simulink model "Sim118Bus"  (R2020b)
(part 2 of 2)

  Branch2-12/RConn1 -- Bus12/RConn1 -- Branch12-12/LConn1 -- Branch12-117/LConn1 -- Branch12-16/LConn1 -- Branch12-14/LConn1 -- Branch11-12/RConn1 -- Branch7-12/RConn1 -- Branch3-12/RConn1
  Branch2-12/RConn2 -- Bus12/RConn2 -- Branch12-12/LConn2 -- Branch12-117/LConn2 -- Branch12-16/LConn2 -- Branch12-14/LConn2 -- Branch11-12/RConn2 -- Branch7-12/RConn2 -- Branch3-12/RConn2
  Branch2-12/RConn3 -- Bus12/RConn3 -- Branch12-12/LConn3 -- Branch12-117/LConn3 -- Branch12-16/LConn3 -- Branch12-14/LConn3 -- Branch11-12/RConn3 -- Branch7-12/RConn3 -- Branch3-12/RConn3
  Branch2-12/LConn1 -- Bus2/RConn1 -- Branch2-2/LConn1 -- Branch2-69/LConn1
  Branch2-12/LConn2 -- Bus2/RConn2 -- Branch2-2/LConn2 -- Branch2-69/LConn2
  Branch2-12/LConn3 -- Bus2/RConn3 -- Branch2-2/LConn3 -- Branch2-69/LConn3
  Branch2-69/RConn1 -- Bus69/RConn1 -- Branch69-69/LConn1 -- Branch3-69/RConn1
  Branch2-69/RConn2 -- Bus69/RConn2 -- Branch69-69/LConn2 -- Branch3-69/RConn2
  Branch2-69/RConn3 -- Bus69/RConn3 -- Branch69-69/LConn3 -- Branch3-69/RConn3
  Branch3-5/RConn1 -- Bus5/RConn1 -- Branch5-5/LConn1 -- Branch5-11/LConn1 -- Transformer5-8/LConn1 -- Branch5-6/LConn1 -- Branch4-5/RConn1
  Branch3-5/RConn2 -- Bus5/RConn2 -- Branch5-5/LConn2 -- Branch5-11/LConn2 -- Transformer5-8/LConn2 -- Branch5-6/LConn2 -- Branch4-5/RConn2
  Branch3-5/RConn3 -- Bus5/RConn3 -- Branch5-5/LConn3 -- Branch5-11/LConn3 -- Transformer5-8/LConn3 -- Branch5-6/LConn3 -- Branch4-5/RConn3
  Branch3-5/LConn1 -- Bus3/RConn1 -- Branch3-3/LConn1 -- Branch3-69/LConn1 -- Branch3-12/LConn1
  Branch3-5/LConn2 -- Bus3/RConn2 -- Branch3-3/LConn2 -- Branch3-69/LConn2 -- Branch3-12/LConn2
  Branch3-5/LConn3 -- Bus3/RConn3 -- Branch3-3/LConn3 -- Branch3-69/LConn3 -- Branch3-12/LConn3
  Branch4-5/LConn1 -- Bus4/RConn1 -- Branch4-4/LConn1 -- Branch4-11/LConn1
  Branch4-5/LConn2 -- Bus4/RConn2 -- Branch4-4/LConn2 -- Branch4-11/LConn2
  Branch4-5/LConn3 -- Bus4/RConn3 -- Branch4-4/LConn3 -- Branch4-11/LConn3
  Branch4-11/RConn1 -- Bus11/RConn1 -- Branch11-11/LConn1 -- Branch11-13/LConn1 -- Branch11-12/LConn1 -- Branch5-11/RConn1
  Branch4-11/RConn2 -- Bus11/RConn2 -- Branch11-11/LConn2 -- Branch11-13/LConn2 -- Branch11-12/LConn2 -- Branch5-11/RConn2
  Branch4-11/RConn3 -- Bus11/RConn3 -- Branch11-11/LConn3 -- Branch11-13/LConn3 -- Branch11-12/LConn3 -- Branch5-11/RConn3
  Branch5-6/RConn1 -- Bus6/RConn1 -- Branch6-6/LConn1 -- Branch6-7/LConn1
  Branch5-6/RConn2 -- Bus6/RConn2 -- Branch6-6/LConn2 -- Branch6-7/LConn2
  Branch5-6/RConn3 -- Bus6/RConn3 -- Branch6-6/LConn3 -- Branch6-7/LConn3
  Branch5-8/RConn1 -- Bus8/RConn1 -- Branch8-8/LConn1 -- Branch8-30/LConn1 -- Branch8-9/LConn1
  Branch5-8/RConn2 -- Bus8/RConn2 -- Branch8-8/LConn2 -- Branch8-30/LConn2 -- Branch8-9/LConn2
  Branch5-8/RConn3 -- Bus8/RConn3 -- Branch8-8/LConn3 -- Branch8-30/LConn3 -- Branch8-9/LConn3
  Transformer5-8/RConn1 -- Branch5-8/LConn1
  Transformer5-8/RConn2 -- Branch5-8/LConn2
  Transformer5-8/RConn3 -- Branch5-8/LConn3
  Branch6-7/RConn1 -- Bus7/RConn1 -- Branch7-7/LConn1 -- Branch7-12/LConn1
  Branch6-7/RConn2 -- Bus7/RConn2 -- Branch7-7/LConn2 -- Branch7-12/LConn2
  Branch6-7/RConn3 -- Bus7/RConn3 -- Branch7-7/LConn3 -- Branch7-12/LConn3
  Branch8-9/RConn1 -- Bus9/RConn1 -- Branch9-9/LConn1 -- Branch9-10/LConn1
  Branch8-9/RConn2 -- Bus9/RConn2 -- Branch9-9/LConn2 -- Branch9-10/LConn2
  Branch8-9/RConn3 -- Bus9/RConn3 -- Branch9-9/LConn3 -- Branch9-10/LConn3
  Branch8-30/RConn1 -- Bus30/RConn1 -- Branch30-30/LConn1 -- Branch30-38/LConn1 -- Branch26-30/RConn1 -- Branch17-30/RConn1
  Branch8-30/RConn2 -- Bus30/RConn2 -- Branch30-30/LConn2 -- Branch30-38/LConn2 -- Branch26-30/RConn2 -- Branch17-30/RConn2
  Branch8-30/RConn3 -- Bus30/RConn3 -- Branch30-30/LConn3 -- Branch30-38/LConn3 -- Branch26-30/RConn3 -- Branch17-30/RConn3
  Branch9-10/RConn1 -- Bus10/RConn1 -- Branch10-10/LConn1
  Branch9-10/RConn2 -- Bus10/RConn2 -- Branch10-10/LConn2
  Branch9-10/RConn3 -- Bus10/RConn3 -- Branch10-10/LConn3
  Branch11-13/RConn1 -- Bus13/RConn1 -- Branch13-13/LConn1 -- Branch13-15/LConn1
  Branch11-13/RConn2 -- Bus13/RConn2 -- Branch13-13/LConn2 -- Branch13-15/LConn2
  Branch11-13/RConn3 -- Bus13/RConn3 -- Branch13-13/LConn3 -- Branch13-15/LConn3
  Branch12-14/RConn1 -- Bus14/RConn1 -- Branch14-14/LConn1 -- Branch14-15/LConn1
  Branch12-14/RConn2 -- Bus14/RConn2 -- Branch14-14/LConn2 -- Branch14-15/LConn2
  Branch12-14/RConn3 -- Bus14/RConn3 -- Branch14-14/LConn3 -- Branch14-15/LConn3
  Branch12-16/RConn1 -- Bus16/RConn1 -- Branch16-16/LConn1 -- Branch16-17/LConn1
  Branch12-16/RConn2 -- Bus16/RConn2 -- Branch16-16/LConn2 -- Branch16-17/LConn2
  Branch12-16/RConn3 -- Bus16/RConn3 -- Branch16-16/LConn3 -- Branch16-17/LConn3
  Branch12-117/RConn1 -- Bus117/RConn1 -- Branch117-117/LConn1
  Branch12-117/RConn2 -- Bus117/RConn2 -- Branch117-117/LConn2
  Branch12-117/RConn3 -- Bus117/RConn3 -- Branch117-117/LConn3
  Branch13-15/RConn1 -- Bus15/RConn1 -- Branch15-15/LConn1 -- Branch15-33/LConn1 -- Branch15-19/LConn1 -- Branch15-17/LConn1 -- Branch14-15/RConn1
  Branch13-15/RConn2 -- Bus15/RConn2 -- Branch15-15/LConn2 -- Branch15-33/LConn2 -- Branch15-19/LConn2 -- Branch15-17/LConn2 -- Branch14-15/RConn2
  Branch13-15/RConn3 -- Bus15/RConn3 -- Branch15-15/LConn3 -- Branch15-33/LConn3 -- Branch15-19/LConn3 -- Branch15-17/LConn3 -- Branch14-15/RConn3
  Branch15-17/RConn1 -- Bus17/RConn1 -- Branch17-17/LConn1 -- Branch17-113/LConn1 -- Branch17-31/LConn1 -- Transformer17-30/LConn1 -- Branch17-18/LConn1 -- Branch16-17/RConn1
  Branch15-17/RConn2 -- Bus17/RConn2 -- Branch17-17/LConn2 -- Branch17-113/LConn2 -- Branch17-31/LConn2 -- Transformer17-30/LConn2 -- Branch17-18/LConn2 -- Branch16-17/RConn2
  Branch15-17/RConn3 -- Bus17/RConn3 -- Branch17-17/LConn3 -- Branch17-113/LConn3 -- Branch17-31/LConn3 -- Transformer17-30/LConn3 -- Branch17-18/LConn3 -- Branch16-17/RConn3
  Branch15-19/RConn1 -- Bus19/RConn1 -- Branch19-19/LConn1 -- Branch19-34/LConn1 -- Branch19-20/LConn1 -- Branch18-19/RConn1
  Branch15-19/RConn2 -- Bus19/RConn2 -- Branch19-19/LConn2 -- Branch19-34/LConn2 -- Branch19-20/LConn2 -- Branch18-19/RConn2
  Branch15-19/RConn3 -- Bus19/RConn3 -- Branch19-19/LConn3 -- Branch19-34/LConn3 -- Branch19-20/LConn3 -- Branch18-19/RConn3
  Branch15-33/RConn1 -- Bus33/RConn1 -- Branch33-33/LConn1 -- Branch33-37/LConn1
  Branch15-33/RConn2 -- Bus33/RConn2 -- Branch33-33/LConn2 -- Branch33-37/LConn2
  Branch15-33/RConn3 -- Bus33/RConn3 -- Branch33-33/LConn3 -- Branch33-37/LConn3
  Branch17-18/RConn1 -- Bus18/RConn1 -- Branch18-18/LConn1 -- Branch18-19/LConn1
  Branch17-18/RConn2 -- Bus18/RConn2 -- Branch18-18/LConn2 -- Branch18-19/LConn2
  Branch17-18/RConn3 -- Bus18/RConn3 -- Branch18-18/LConn3 -- Branch18-19/LConn3
  Transformer17-30/RConn1 -- Branch17-30/LConn1
  Transformer17-30/RConn2 -- Branch17-30/LConn2
  Transformer17-30/RConn3 -- Branch17-30/LConn3
  Branch17-31/RConn1 -- Bus31/RConn1 -- Branch31-31/LConn1 -- Branch31-32/LConn1 -- Branch29-31/RConn1
  Branch17-31/RConn2 -- Bus31/RConn2 -- Branch31-31/LConn2 -- Branch31-32/LConn2 -- Branch29-31/RConn2
  Branch17-31/RConn3 -- Bus31/RConn3 -- Branch31-31/LConn3 -- Branch31-32/LConn3 -- Branch29-31/RConn3
  Branch17-113/RConn1 -- Bus113/RConn1 -- Branch113-113/LConn1 -- Branch32-113/RConn1
  Branch17-113/RConn2 -- Bus113/RConn2 -- Branch113-113/LConn2 -- Branch32-113/RConn2
  Branch17-113/RConn3 -- Bus113/RConn3 -- Branch113-113/LConn3 -- Branch32-113/RConn3
  Branch19-20/RConn1 -- Bus20/RConn1 -- Branch20-20/LConn1 -- Branch20-21/LConn1
  Branch19-20/RConn2 -- Bus20/RConn2 -- Branch20-20/LConn2 -- Branch20-21/LConn2
  Branch19-20/RConn3 -- Bus20/RConn3 -- Branch20-20/LConn3 -- Branch20-21/LConn3
  Branch19-34/RConn1 -- Bus34/RConn1 -- Branch34-34/LConn1 -- Branch34-43/LConn1 -- Branch34-37/LConn1 -- Branch34-36/LConn1
  Branch19-34/RConn2 -- Bus34/RConn2 -- Branch34-34/LConn2 -- Branch34-43/LConn2 -- Branch34-37/LConn2 -- Branch34-36/LConn2
  Branch19-34/RConn3 -- Bus34/RConn3 -- Branch34-34/LConn3 -- Branch34-43/LConn3 -- Branch34-37/LConn3 -- Branch34-36/LConn3
  Branch20-21/RConn1 -- Bus21/RConn1 -- Branch21-21/LConn1 -- Branch21-22/LConn1
  Branch20-21/RConn2 -- Bus21/RConn2 -- Branch21-21/LConn2 -- Branch21-22/LConn2
  Branch20-21/RConn3 -- Bus21/RConn3 -- Branch21-21/LConn3 -- Branch21-22/LConn3
  Branch21-22/RConn1 -- Bus22/RConn1 -- Branch22-22/LConn1 -- Branch22-23/LConn1
  Branch21-22/RConn2 -- Bus22/RConn2 -- Branch22-22/LConn2 -- Branch22-23/LConn2
  Branch21-22/RConn3 -- Bus22/RConn3 -- Branch22-22/LConn3 -- Branch22-23/LConn3
  Branch22-23/RConn1 -- Bus23/RConn1 -- Branch23-23/LConn1 -- Branch23-32/LConn1 -- Branch23-25/LConn1 -- Branch23-24/LConn1
  Branch22-23/RConn2 -- Bus23/RConn2 -- Branch23-23/LConn2 -- Branch23-32/LConn2 -- Branch23-25/LConn2 -- Branch23-24/LConn2
  Branch22-23/RConn3 -- Bus23/RConn3 -- Branch23-23/LConn3 -- Branch23-32/LConn3 -- Branch23-25/LConn3 -- Branch23-24/LConn3
  Branch23-24/RConn1 -- Bus24/RConn1 -- Branch24-24/LConn1 -- Branch24-72/LConn1 -- Branch24-70/LConn1
  Branch23-24/RConn2 -- Bus24/RConn2 -- Branch24-24/LConn2 -- Branch24-72/LConn2 -- Branch24-70/LConn2
  Branch23-24/RConn3 -- Bus24/RConn3 -- Branch24-24/LConn3 -- Branch24-72/LConn3 -- Branch24-70/LConn3
  Branch23-25/RConn1 -- Bus25/RConn1 -- Branch25-25/LConn1 -- Branch25-27/LConn1 -- Transformer25-26/LConn1
  Branch23-25/RConn2 -- Bus25/RConn2 -- Branch25-25/LConn2 -- Branch25-27/LConn2 -- Transformer25-26/LConn2
  Branch23-25/RConn3 -- Bus25/RConn3 -- Branch25-25/LConn3 -- Branch25-27/LConn3 -- Transformer25-26/LConn3
  Branch23-32/RConn1 -- Bus32/RConn1 -- Branch32-32/LConn1 -- Branch32-114/LConn1 -- Branch32-113/LConn1 -- Branch31-32/RConn1 -- Branch27-32/RConn1
  Branch23-32/RConn2 -- Bus32/RConn2 -- Branch32-32/LConn2 -- Branch32-114/LConn2 -- Branch32-113/LConn2 -- Branch31-32/RConn2 -- Branch27-32/RConn2
  Branch23-32/RConn3 -- Bus32/RConn3 -- Branch32-32/LConn3 -- Branch32-114/LConn3 -- Branch32-113/LConn3 -- Branch31-32/RConn3 -- Branch27-32/RConn3
  Branch24-72/RConn1 -- Bus72/RConn1 -- Branch72-72/LConn1 -- Branch71-72/RConn1
  Branch24-72/RConn2 -- Bus72/RConn2 -- Branch72-72/LConn2 -- Branch71-72/RConn2
  Branch24-72/RConn3 -- Bus72/RConn3 -- Branch72-72/LConn3 -- Branch71-72/RConn3
  Branch25-26/RConn1 -- Bus26/RConn1 -- Branch26-26/LConn1 -- Branch26-30/LConn1
  Branch25-26/RConn2 -- Bus26/RConn2 -- Branch26-26/LConn2 -- Branch26-30/LConn2
  Branch25-26/RConn3 -- Bus26/RConn3 -- Branch26-26/LConn3 -- Branch26-30/LConn3
  Transformer25-26/RConn1 -- Branch25-26/LConn1
  Transformer25-26/RConn2 -- Branch25-26/LConn2
  Transformer25-26/RConn3 -- Branch25-26/LConn3
  Branch25-27/RConn1 -- Bus27/RConn1 -- Branch27-27/LConn1 -- Branch27-115/LConn1 -- Branch27-32/LConn1 -- Branch27-28/LConn1
  Branch25-27/RConn2 -- Bus27/RConn2 -- Branch27-27/LConn2 -- Branch27-115/LConn2 -- Branch27-32/LConn2 -- Branch27-28/LConn2
  Branch25-27/RConn3 -- Bus27/RConn3 -- Branch27-27/LConn3 -- Branch27-115/LConn3 -- Branch27-32/LConn3 -- Branch27-28/LConn3
  Branch27-28/RConn1 -- Bus28/RConn1 -- Branch28-28/LConn1 -- Branch28-29/LConn1
  Branch27-28/RConn2 -- Bus28/RConn2 -- Branch28-28/LConn2 -- Branch28-29/LConn2
  Branch27-28/RConn3 -- Bus28/RConn3 -- Branch28-28/LConn3 -- Branch28-29/LConn3
  Branch27-115/RConn1 -- Bus115/RConn1 -- Branch115-115/LConn1 -- Branch114-115/RConn1
  Branch27-115/RConn2 -- Bus115/RConn2 -- Branch115-115/LConn2 -- Branch114-115/RConn2
  Branch27-115/RConn3 -- Bus115/RConn3 -- Branch115-115/LConn3 -- Branch114-115/RConn3
  Branch28-29/RConn1 -- Bus29/RConn1 -- Branch29-29/LConn1 -- Branch29-31/LConn1
  Branch28-29/RConn2 -- Bus29/RConn2 -- Branch29-29/LConn2 -- Branch29-31/LConn2
  Branch28-29/RConn3 -- Bus29/RConn3 -- Branch29-29/LConn3 -- Branch29-31/LConn3
  Branch30-38/RConn1 -- Bus38/RConn1 -- Branch38-38/LConn1 -- Branch38-65/LConn1 -- Branch37-38/RConn1
  Branch30-38/RConn2 -- Bus38/RConn2 -- Branch38-38/LConn2 -- Branch38-65/LConn2 -- Branch37-38/RConn2
  Branch30-38/RConn3 -- Bus38/RConn3 -- Branch38-38/LConn3 -- Branch38-65/LConn3 -- Branch37-38/RConn3
  Branch32-114/RConn1 -- Bus114/RConn1 -- Branch114-114/LConn1 -- Branch114-115/LConn1
  Branch32-114/RConn2 -- Bus114/RConn2 -- Branch114-114/LConn2 -- Branch114-115/LConn2
  Branch32-114/RConn3 -- Bus114/RConn3 -- Branch114-114/LConn3 -- Branch114-115/LConn3
  Branch33-37/RConn1 -- Bus37/RConn1 -- Branch37-37/LConn1 -- Branch37-40/LConn1 -- Branch37-39/LConn1 -- Transformer37-38/LConn1 -- Branch35-37/RConn1 -- Branch34-37/RConn1
  Branch33-37/RConn2 -- Bus37/RConn2 -- Branch37-37/LConn2 -- Branch37-40/LConn2 -- Branch37-39/LConn2 -- Transformer37-38/LConn2 -- Branch35-37/RConn2 -- Branch34-37/RConn2
  Branch33-37/RConn3 -- Bus37/RConn3 -- Branch37-37/LConn3 -- Branch37-40/LConn3 -- Branch37-39/LConn3 -- Transformer37-38/LConn3 -- Branch35-37/RConn3 -- Branch34-37/RConn3
  Branch34-36/RConn1 -- Bus36/RConn1 -- Branch36-36/LConn1 -- Branch35-36/RConn1
  Branch34-36/RConn2 -- Bus36/RConn2 -- Branch36-36/LConn2 -- Branch35-36/RConn2
  Branch34-36/RConn3 -- Bus36/RConn3 -- Branch36-36/LConn3 -- Branch35-36/RConn3
  Branch34-43/RConn1 -- Bus43/RConn1 -- Branch43-43/LConn1 -- Branch43-44/LConn1
  Branch34-43/RConn2 -- Bus43/RConn2 -- Branch43-43/LConn2 -- Branch43-44/LConn2
  Branch34-43/RConn3 -- Bus43/RConn3 -- Branch43-43/LConn3 -- Branch43-44/LConn3
  Branch35-36/LConn1 -- Bus35/RConn1 -- Branch35-35/LConn1 -- Branch35-37/LConn1
  Branch35-36/LConn2 -- Bus35/RConn2 -- Branch35-35/LConn2 -- Branch35-37/LConn2
  Branch35-36/LConn3 -- Bus35/RConn3 -- Branch35-35/LConn3 -- Branch35-37/LConn3
  Transformer37-38/RConn1 -- Branch37-38/LConn1
  Transformer37-38/RConn2 -- Branch37-38/LConn2
  Transformer37-38/RConn3 -- Branch37-38/LConn3
  Branch37-39/RConn1 -- Bus39/RConn1 -- Branch39-39/LConn1 -- Branch39-40/LConn1
  Branch37-39/RConn2 -- Bus39/RConn2 -- Branch39-39/LConn2 -- Branch39-40/LConn2
  Branch37-39/RConn3 -- Bus39/RConn3 -- Branch39-39/LConn3 -- Branch39-40/LConn3
  Branch37-40/RConn1 -- Bus40/RConn1 -- Branch40-40/LConn1 -- Branch40-42/LConn1 -- Branch40-41/LConn1 -- Branch39-40/RConn1
  Branch37-40/RConn2 -- Bus40/RConn2 -- Branch40-40/LConn2 -- Branch40-42/LConn2 -- Branch40-41/LConn2 -- Branch39-40/RConn2
  Branch37-40/RConn3 -- Bus40/RConn3 -- Branch40-40/LConn3 -- Branch40-42/LConn3 -- Branch40-41/LConn3 -- Branch39-40/RConn3
  Branch38-65/RConn1 -- Bus65/RConn1 -- Branch65-65/LConn1 -- Branch65-68/LConn1 -- Transformer65-66/LConn1 -- Branch64-65/RConn1
  Branch38-65/RConn2 -- Bus65/RConn2 -- Branch65-65/LConn2 -- Branch65-68/LConn2 -- Transformer65-66/LConn2 -- Branch64-65/RConn2
  Branch38-65/RConn3 -- Bus65/RConn3 -- Branch65-65/LConn3 -- Branch65-68/LConn3 -- Transformer65-66/LConn3 -- Branch64-65/RConn3
  Branch40-41/RConn1 -- Bus41/RConn1 -- Branch41-41/LConn1 -- Branch41-42/LConn1
  Branch40-41/RConn2 -- Bus41/RConn2 -- Branch41-41/LConn2 -- Branch41-42/LConn2
  Branch40-41/RConn3 -- Bus41/RConn3 -- Branch41-41/LConn3 -- Branch41-42/LConn3
  Branch40-42/RConn1 -- Bus42/RConn1 -- Branch42-42/LConn1 -- Branch42-49_/LConn1 -- Branch42-49/LConn1 -- Branch41-42/RConn1
  Branch40-42/RConn2 -- Bus42/RConn2 -- Branch42-42/LConn2 -- Branch42-49_/LConn2 -- Branch42-49/LConn2 -- Branch41-42/RConn2
  Branch40-42/RConn3 -- Bus42/RConn3 -- Branch42-42/LConn3 -- Branch42-49_/LConn3 -- Branch42-49/LConn3 -- Branch41-42/RConn3
  Branch43-44/RConn1 -- Bus44/RConn1 -- Branch44-44/LConn1 -- Branch44-45/LConn1
  Branch43-44/RConn2 -- Bus44/RConn2 -- Branch44-44/LConn2 -- Branch44-45/LConn2
  Branch43-44/RConn3 -- Bus44/RConn3 -- Branch44-44/LConn3 -- Branch44-45/LConn3
  Branch44-45/RConn1 -- Bus45/RConn1 -- Branch45-45/LConn1 -- Branch45-49/LConn1 -- Branch45-46/LConn1
  Branch44-45/RConn2 -- Bus45/RConn2 -- Branch45-45/LConn2 -- Branch45-49/LConn2 -- Branch45-46/LConn2
  Branch44-45/RConn3 -- Bus45/RConn3 -- Branch45-45/LConn3 -- Branch45-49/LConn3 -- Branch45-46/LConn3
  Branch45-46/RConn1 -- Bus46/RConn1 -- Branch46-46/LConn1 -- Branch46-48/LConn1 -- Branch46-47/LConn1
  Branch45-46/RConn2 -- Bus46/RConn2 -- Branch46-46/LConn2 -- Branch46-48/LConn2 -- Branch46-47/LConn2
  Branch45-46/RConn3 -- Bus46/RConn3 -- Branch46-46/LConn3 -- Branch46-48/LConn3 -- Branch46-47/LConn3
  Branch46-48/RConn1 -- Bus48/RConn1 -- Branch48-48/LConn1 -- Branch48-49/LConn1
  Branch46-48/RConn2 -- Bus48/RConn2 -- Branch48-48/LConn2 -- Branch48-49/LConn2
  Branch46-48/RConn3 -- Bus48/RConn3 -- Branch48-48/LConn3 -- Branch48-49/LConn3
  Branch49-50/RConn1 -- Bus50/RConn1 -- Branch50-50/LConn1 -- Branch50-57/LConn1
  Branch49-50/RConn2 -- Bus50/RConn2 -- Branch50-50/LConn2 -- Branch50-57/LConn2
  Branch49-50/RConn3 -- Bus50/RConn3 -- Branch50-50/LConn3 -- Branch50-57/LConn3
  Branch49-51/RConn1 -- Bus51/RConn1 -- Branch51-51/LConn1 -- Branch51-58/LConn1 -- Branch51-52/LConn1
  Branch49-51/RConn2 -- Bus51/RConn2 -- Branch51-51/LConn2 -- Branch51-58/LConn2 -- Branch51-52/LConn2
  Branch49-51/RConn3 -- Bus51/RConn3 -- Branch51-51/LConn3 -- Branch51-58/LConn3 -- Branch51-52/LConn3
  Branch49-54/RConn1 -- Bus54/RConn1 -- Branch54-54/LConn1 -- Branch54-59/LConn1 -- Branch54-56/LConn1 -- Branch54-55/LConn1 -- Branch53-54/RConn1 -- Branch49-54_/RConn1
  Branch49-54/RConn2 -- Bus54/RConn2 -- Branch54-54/LConn2 -- Branch54-59/LConn2 -- Branch54-56/LConn2 -- Branch54-55/LConn2 -- Branch53-54/RConn2 -- Branch49-54_/RConn2
  Branch49-54/RConn3 -- Bus54/RConn3 -- Branch54-54/LConn3 -- Branch54-59/LConn3 -- Branch54-56/LConn3 -- Branch54-55/LConn3 -- Branch53-54/RConn3 -- Branch49-54_/RConn3
  Branch49-66/RConn1 -- Bus66/RConn1 -- Branch66-66/LConn1 -- Branch66-67/LConn1 -- Branch65-66/RConn1 -- Branch62-66/RConn1 -- Branch49-66_/RConn1
  Branch49-66/RConn2 -- Bus66/RConn2 -- Branch66-66/LConn2 -- Branch66-67/LConn2 -- Branch65-66/RConn2 -- Branch62-66/RConn2 -- Branch49-66_/RConn2
  Branch49-66/RConn3 -- Bus66/RConn3 -- Branch66-66/LConn3 -- Branch66-67/LConn3 -- Branch65-66/RConn3 -- Branch62-66/RConn3 -- Branch49-66_/RConn3
  Branch50-57/RConn1 -- Bus57/RConn1 -- Branch57-57/LConn1 -- Branch56-57/RConn1
  Branch50-57/RConn2 -- Bus57/RConn2 -- Branch57-57/LConn2 -- Branch56-57/RConn2
  Branch50-57/RConn3 -- Bus57/RConn3 -- Branch57-57/LConn3 -- Branch56-57/RConn3
  Branch51-52/RConn1 -- Bus52/RConn1 -- Branch52-52/LConn1 -- Branch52-53/LConn1
  Branch51-52/RConn2 -- Bus52/RConn2 -- Branch52-52/LConn2 -- Branch52-53/LConn2
  Branch51-52/RConn3 -- Bus52/RConn3 -- Branch52-52/LConn3 -- Branch52-53/LConn3
  Branch51-58/RConn1 -- Bus58/RConn1 -- Branch58-58/LConn1 -- Branch56-58/RConn1
  Branch51-58/RConn2 -- Bus58/RConn2 -- Branch58-58/LConn2 -- Branch56-58/RConn2
  Branch51-58/RConn3 -- Bus58/RConn3 -- Branch58-58/LConn3 -- Branch56-58/RConn3
  Branch52-53/RConn1 -- Bus53/RConn1 -- Branch53-53/LConn1 -- Branch53-54/LConn1
  Branch52-53/RConn2 -- Bus53/RConn2 -- Branch53-53/LConn2 -- Branch53-54/LConn2
  Branch52-53/RConn3 -- Bus53/RConn3 -- Branch53-53/LConn3 -- Branch53-54/LConn3
  Branch54-55/RConn1 -- Bus55/RConn1 -- Branch55-55/LConn1 -- Branch55-59/LConn1 -- Branch55-56/LConn1
  Branch54-55/RConn2 -- Bus55/RConn2 -- Branch55-55/LConn2 -- Branch55-59/LConn2 -- Branch55-56/LConn2
  Branch54-55/RConn3 -- Bus55/RConn3 -- Branch55-55/LConn3 -- Branch55-59/LConn3 -- Branch55-56/LConn3
  Branch54-56/RConn1 -- Bus56/RConn1 -- Branch56-56/LConn1 -- Branch56-59_/LConn1 -- Branch56-59/LConn1 -- Branch56-58/LConn1 -- Branch56-57/LConn1 -- Branch55-56/RConn1
  Branch54-56/RConn2 -- Bus56/RConn2 -- Branch56-56/LConn2 -- Branch56-59_/LConn2 -- Branch56-59/LConn2 -- Branch56-58/LConn2 -- Branch56-57/LConn2 -- Branch55-56/RConn2
  Branch54-56/RConn3 -- Bus56/RConn3 -- Branch56-56/LConn3 -- Branch56-59_/LConn3 -- Branch56-59/LConn3 -- Branch56-58/LConn3 -- Branch56-57/LConn3 -- Branch55-56/RConn3
  Branch54-59/RConn1 -- Bus59/RConn1 -- Branch59-59/LConn1 -- Transformer59-63/LConn1 -- Branch59-61/LConn1 -- Branch59-60/LConn1 -- Branch56-59_/RConn1 -- Branch56-59/RConn1 -- Branch55-59/RConn1
  Branch54-59/RConn2 -- Bus59/RConn2 -- Branch59-59/LConn2 -- Transformer59-63/LConn2 -- Branch59-61/LConn2 -- Branch59-60/LConn2 -- Branch56-59_/RConn2 -- Branch56-59/RConn2 -- Branch55-59/RConn2
  Branch54-59/RConn3 -- Bus59/RConn3 -- Branch59-59/LConn3 -- Transformer59-63/LConn3 -- Branch59-61/LConn3 -- Branch59-60/LConn3 -- Branch56-59_/RConn3 -- Branch56-59/RConn3 -- Branch55-59/RConn3
  Branch59-60/RConn1 -- Bus60/RConn1 -- Branch60-60/LConn1 -- Branch60-62/LConn1 -- Branch60-61/LConn1
  Branch59-60/RConn2 -- Bus60/RConn2 -- Branch60-60/LConn2 -- Branch60-62/LConn2 -- Branch60-61/LConn2
  Branch59-60/RConn3 -- Bus60/RConn3 -- Branch60-60/LConn3 -- Branch60-62/LConn3 -- Branch60-61/LConn3
  Branch59-61/RConn1 -- Bus61/RConn1 -- Branch61-61/LConn1 -- Transformer61-64/LConn1 -- Branch61-62/LConn1 -- Branch60-61/RConn1
  Branch59-61/RConn2 -- Bus61/RConn2 -- Branch61-61/LConn2 -- Transformer61-64/LConn2 -- Branch61-62/LConn2 -- Branch60-61/RConn2
  Branch59-61/RConn3 -- Bus61/RConn3 -- Branch61-61/LConn3 -- Transformer61-64/LConn3 -- Branch61-62/LConn3 -- Branch60-61/RConn3
  Branch59-63/RConn1 -- Bus63/RConn1 -- Branch63-63/LConn1 -- Branch63-64/LConn1
  Branch59-63/RConn2 -- Bus63/RConn2 -- Branch63-63/LConn2 -- Branch63-64/LConn2
  Branch59-63/RConn3 -- Bus63/RConn3 -- Branch63-63/LConn3 -- Branch63-64/LConn3
  Transformer59-63/RConn1 -- Branch59-63/LConn1
  Transformer59-63/RConn2 -- Branch59-63/LConn2
  Transformer59-63/RConn3 -- Branch59-63/LConn3
  Branch60-62/RConn1 -- Bus62/RConn1 -- Branch62-62/LConn1 -- Branch62-67/LConn1 -- Branch62-66/LConn1 -- Branch61-62/RConn1
  Branch60-62/RConn2 -- Bus62/RConn2 -- Branch62-62/LConn2 -- Branch62-67/LConn2 -- Branch62-66/LConn2 -- Branch61-62/RConn2
  Branch60-62/RConn3 -- Bus62/RConn3 -- Branch62-62/LConn3 -- Branch62-67/LConn3 -- Branch62-66/LConn3 -- Branch61-62/RConn3
  Branch61-64/RConn1 -- Bus64/RConn1 -- Branch64-64/LConn1 -- Branch64-65/LConn1 -- Branch63-64/RConn1
  Branch61-64/RConn2 -- Bus64/RConn2 -- Branch64-64/LConn2 -- Branch64-65/LConn2 -- Branch63-64/RConn2
  Branch61-64/RConn3 -- Bus64/RConn3 -- Branch64-64/LConn3 -- Branch64-65/LConn3 -- Branch63-64/RConn3
  Transformer61-64/RConn1 -- Branch61-64/LConn1
  Transformer61-64/RConn2 -- Branch61-64/LConn2
  Transformer61-64/RConn3 -- Branch61-64/LConn3
  Branch62-67/RConn1 -- Bus67/RConn1 -- Branch67-67/LConn1 -- Branch66-67/RConn1
  Branch62-67/RConn2 -- Bus67/RConn2 -- Branch67-67/LConn2 -- Branch66-67/RConn2
  Branch62-67/RConn3 -- Bus67/RConn3 -- Branch67-67/LConn3 -- Branch66-67/RConn3
  Transformer65-66/RConn1 -- Branch65-66/LConn1
  Transformer65-66/RConn2 -- Branch65-66/LConn2
  Transformer65-66/RConn3 -- Branch65-66/LConn3
  Branch68-81/RConn1 -- Bus81/RConn1 -- Branch81-81/LConn1 -- Branch80-81/RConn1
  Branch68-81/RConn2 -- Bus81/RConn2 -- Branch81-81/LConn2 -- Branch80-81/RConn2
  Branch68-81/RConn3 -- Bus81/RConn3 -- Branch81-81/LConn3 -- Branch80-81/RConn3
  Branch68-116/RConn1 -- Bus116/RConn1 -- Branch116-116/LConn1
  Branch68-116/RConn2 -- Bus116/RConn2 -- Branch116-116/LConn2
  Branch68-116/RConn3 -- Bus116/RConn3 -- Branch116-116/LConn3
  Branch70-71/RConn1 -- Bus71/RConn1 -- Branch71-71/LConn1 -- Branch71-73/LConn1 -- Branch71-72/LConn1
  Branch70-71/RConn2 -- Bus71/RConn2 -- Branch71-71/LConn2 -- Branch71-73/LConn2 -- Branch71-72/LConn2
  Branch70-71/RConn3 -- Bus71/RConn3 -- Branch71-71/LConn3 -- Branch71-73/LConn3 -- Branch71-72/LConn3
  Branch70-74/RConn1 -- Bus74/RConn1 -- Branch74-74/LConn1 -- Branch74-75/LConn1
  Branch70-74/RConn2 -- Bus74/RConn2 -- Branch74-74/LConn2 -- Branch74-75/LConn2
  Branch70-74/RConn3 -- Bus74/RConn3 -- Branch74-74/LConn3 -- Branch74-75/LConn3
  Branch71-73/RConn1 -- Bus73/RConn1 -- Branch73-73/LConn1
  Branch71-73/RConn2 -- Bus73/RConn2 -- Branch73-73/LConn2
  Branch71-73/RConn3 -- Bus73/RConn3 -- Branch73-73/LConn3
  Branch75-118/RConn1 -- Bus118/RConn1 -- Branch118-118/LConn1 -- Branch76-118/RConn1
  Branch75-118/RConn2 -- Bus118/RConn2 -- Branch118-118/LConn2 -- Branch76-118/RConn2
  Branch75-118/RConn3 -- Bus118/RConn3 -- Branch118-118/LConn3 -- Branch76-118/RConn3
  Branch76-77/LConn1 -- Bus76/RConn1 -- Branch76-76/LConn1 -- Branch76-118/LConn1
  Branch76-77/LConn2 -- Bus76/RConn2 -- Branch76-76/LConn2 -- Branch76-118/LConn2
  Branch76-77/LConn3 -- Bus76/RConn3 -- Branch76-76/LConn3 -- Branch76-118/LConn3
  Branch77-78/RConn1 -- Bus78/RConn1 -- Branch78-78/LConn1 -- Branch78-79/LConn1
  Branch77-78/RConn2 -- Bus78/RConn2 -- Branch78-78/LConn2 -- Branch78-79/LConn2
  Branch77-78/RConn3 -- Bus78/RConn3 -- Branch78-78/LConn3 -- Branch78-79/LConn3
  Branch77-80/RConn1 -- Bus80/RConn1 -- Branch80-80/LConn1 -- Branch80-99/LConn1 -- Branch80-98/LConn1 -- Branch80-97/LConn1 -- Branch80-96/LConn1 -- Transformer80-81/LConn1 -- Branch79-80/RConn1 -- Branch77-80_/RConn1
  Branch77-80/RConn2 -- Bus80/RConn2 -- Branch80-80/LConn2 -- Branch80-99/LConn2 -- Branch80-98/LConn2 -- Branch80-97/LConn2 -- Branch80-96/LConn2 -- Transformer80-81/LConn2 -- Branch79-80/RConn2 -- Branch77-80_/RConn2
  Branch77-80/RConn3 -- Bus80/RConn3 -- Branch80-80/LConn3 -- Branch80-99/LConn3 -- Branch80-98/LConn3 -- Branch80-97/LConn3 -- Branch80-96/LConn3 -- Transformer80-81/LConn3 -- Branch79-80/RConn3 -- Branch77-80_/RConn3
  Branch77-82/RConn1 -- Bus82/RConn1 -- Branch82-82/LConn1 -- Branch82-96/LConn1 -- Branch82-83/LConn1
  Branch77-82/RConn2 -- Bus82/RConn2 -- Branch82-82/LConn2 -- Branch82-96/LConn2 -- Branch82-83/LConn2
  Branch77-82/RConn3 -- Bus82/RConn3 -- Branch82-82/LConn3 -- Branch82-96/LConn3 -- Branch82-83/LConn3
  Branch78-79/RConn1 -- Bus79/RConn1 -- Branch79-79/LConn1 -- Branch79-80/LConn1
  Branch78-79/RConn2 -- Bus79/RConn2 -- Branch79-79/LConn2 -- Branch79-80/LConn2
  Branch78-79/RConn3 -- Bus79/RConn3 -- Branch79-79/LConn3 -- Branch79-80/LConn3
  Transformer80-81/RConn1 -- Branch80-81/LConn1
  Transformer80-81/RConn2 -- Branch80-81/LConn2
  Transformer80-81/RConn3 -- Branch80-81/LConn3
  Branch80-96/RConn1 -- Bus96/RConn1 -- Branch96-96/LConn1 -- Branch96-97/LConn1 -- Branch95-96/RConn1 -- Branch94-96/RConn1 -- Branch82-96/RConn1
  Branch80-96/RConn2 -- Bus96/RConn2 -- Branch96-96/LConn2 -- Branch96-97/LConn2 -- Branch95-96/RConn2 -- Branch94-96/RConn2 -- Branch82-96/RConn2
  Branch80-96/RConn3 -- Bus96/RConn3 -- Branch96-96/LConn3 -- Branch96-97/LConn3 -- Branch95-96/RConn3 -- Branch94-96/RConn3 -- Branch82-96/RConn3
  Branch80-97/RConn1 -- Bus97/RConn1 -- Branch97-97/LConn1 -- Branch96-97/RConn1
  Branch80-97/RConn2 -- Bus97/RConn2 -- Branch97-97/LConn2 -- Branch96-97/RConn2
  Branch80-97/RConn3 -- Bus97/RConn3 -- Branch97-97/LConn3 -- Branch96-97/RConn3
  Branch80-98/RConn1 -- Bus98/RConn1 -- Branch98-98/LConn1 -- Branch98-100/LConn1
  Branch80-98/RConn2 -- Bus98/RConn2 -- Branch98-98/LConn2 -- Branch98-100/LConn2
  Branch80-98/RConn3 -- Bus98/RConn3 -- Branch98-98/LConn3 -- Branch98-100/LConn3
  Branch80-99/RConn1 -- Bus99/RConn1 -- Branch99-99/LConn1 -- Branch99-100/LConn1
  Branch80-99/RConn2 -- Bus99/RConn2 -- Branch99-99/LConn2 -- Branch99-100/LConn2
  Branch80-99/RConn3 -- Bus99/RConn3 -- Branch99-99/LConn3 -- Branch99-100/LConn3
  Branch82-83/RConn1 -- Bus83/RConn1 -- Branch83-83/LConn1 -- Branch83-85/LConn1 -- Branch83-84/LConn1
  Branch82-83/RConn2 -- Bus83/RConn2 -- Branch83-83/LConn2 -- Branch83-85/LConn2 -- Branch83-84/LConn2
  Branch82-83/RConn3 -- Bus83/RConn3 -- Branch83-83/LConn3 -- Branch83-85/LConn3 -- Branch83-84/LConn3
  Branch83-84/RConn1 -- Bus84/RConn1 -- Branch84-84/LConn1 -- Branch84-85/LConn1
  Branch83-84/RConn2 -- Bus84/RConn2 -- Branch84-84/LConn2 -- Branch84-85/LConn2
  Branch83-84/RConn3 -- Bus84/RConn3 -- Branch84-84/LConn3 -- Branch84-85/LConn3
  Branch83-85/RConn1 -- Bus85/RConn1 -- Branch85-85/LConn1 -- Branch85-89/LConn1 -- Branch85-88/LConn1 -- Branch85-86/LConn1 -- Branch84-85/RConn1
  Branch83-85/RConn2 -- Bus85/RConn2 -- Branch85-85/LConn2 -- Branch85-89/LConn2 -- Branch85-88/LConn2 -- Branch85-86/LConn2 -- Branch84-85/RConn2
  Branch83-85/RConn3 -- Bus85/RConn3 -- Branch85-85/LConn3 -- Branch85-89/LConn3 -- Branch85-88/LConn3 -- Branch85-86/LConn3 -- Branch84-85/RConn3
  Branch85-86/RConn1 -- Bus86/RConn1 -- Branch86-86/LConn1 -- Branch86-87/LConn1
  Branch85-86/RConn2 -- Bus86/RConn2 -- Branch86-86/LConn2 -- Branch86-87/LConn2
  Branch85-86/RConn3 -- Bus86/RConn3 -- Branch86-86/LConn3 -- Branch86-87/LConn3
  Branch85-88/RConn1 -- Bus88/RConn1 -- Branch88-88/LConn1 -- Branch88-89/LConn1
  Branch85-88/RConn2 -- Bus88/RConn2 -- Branch88-88/LConn2 -- Branch88-89/LConn2
  Branch85-88/RConn3 -- Bus88/RConn3 -- Branch88-88/LConn3 -- Branch88-89/LConn3
  Branch85-89/RConn1 -- Bus89/RConn1 -- Branch89-89/LConn1 -- Branch89-92_/LConn1 -- Branch89-92/LConn1 -- Branch89-90_/LConn1 -- Branch89-90/LConn1 -- Branch88-89/RConn1
  Branch85-89/RConn2 -- Bus89/RConn2 -- Branch89-89/LConn2 -- Branch89-92_/LConn2 -- Branch89-92/LConn2 -- Branch89-90_/LConn2 -- Branch89-90/LConn2 -- Branch88-89/RConn2
  Branch85-89/RConn3 -- Bus89/RConn3 -- Branch89-89/LConn3 -- Branch89-92_/LConn3 -- Branch89-92/LConn3 -- Branch89-90_/LConn3 -- Branch89-90/LConn3 -- Branch88-89/RConn3
  Branch86-87/RConn1 -- Bus87/RConn1 -- Branch87-87/LConn1
  Branch86-87/RConn2 -- Bus87/RConn2 -- Branch87-87/LConn2
  Branch86-87/RConn3 -- Bus87/RConn3 -- Branch87-87/LConn3
  Branch89-90/RConn1 -- Bus90/RConn1 -- Branch90-90/LConn1 -- Branch90-91/LConn1 -- Branch89-90_/RConn1
  Branch89-90/RConn2 -- Bus90/RConn2 -- Branch90-90/LConn2 -- Branch90-91/LConn2 -- Branch89-90_/RConn2
  Branch89-90/RConn3 -- Bus90/RConn3 -- Branch90-90/LConn3 -- Branch90-91/LConn3 -- Branch89-90_/RConn3
  Branch89-92/RConn1 -- Bus92/RConn1 -- Branch92-92/LConn1 -- Branch92-102/LConn1 -- Branch92-100/LConn1 -- Branch92-94/LConn1 -- Branch92-93/LConn1 -- Branch91-92/RConn1 -- Branch89-92_/RConn1
  Branch89-92/RConn2 -- Bus92/RConn2 -- Branch92-92/LConn2 -- Branch92-102/LConn2 -- Branch92-100/LConn2 -- Branch92-94/LConn2 -- Branch92-93/LConn2 -- Branch91-92/RConn2 -- Branch89-92_/RConn2
  Branch89-92/RConn3 -- Bus92/RConn3 -- Branch92-92/LConn3 -- Branch92-102/LConn3 -- Branch92-100/LConn3 -- Branch92-94/LConn3 -- Branch92-93/LConn3 -- Branch91-92/RConn3 -- Branch89-92_/RConn3
  Branch90-91/RConn1 -- Bus91/RConn1 -- Branch91-91/LConn1 -- Branch91-92/LConn1
  Branch90-91/RConn2 -- Bus91/RConn2 -- Branch91-91/LConn2 -- Branch91-92/LConn2
  Branch90-91/RConn3 -- Bus91/RConn3 -- Branch91-91/LConn3 -- Branch91-92/LConn3
  Branch92-93/RConn1 -- Bus93/RConn1 -- Branch93-93/LConn1 -- Branch93-94/LConn1
  Branch92-93/RConn2 -- Bus93/RConn2 -- Branch93-93/LConn2 -- Branch93-94/LConn2
  Branch92-93/RConn3 -- Bus93/RConn3 -- Branch93-93/LConn3 -- Branch93-94/LConn3
  Branch92-94/RConn1 -- Bus94/RConn1 -- Branch94-94/LConn1 -- Branch94-100/LConn1 -- Branch94-96/LConn1 -- Branch94-95/LConn1 -- Branch93-94/RConn1
  Branch92-94/RConn2 -- Bus94/RConn2 -- Branch94-94/LConn2 -- Branch94-100/LConn2 -- Branch94-96/LConn2 -- Branch94-95/LConn2 -- Branch93-94/RConn2
  Branch92-94/RConn3 -- Bus94/RConn3 -- Branch94-94/LConn3 -- Branch94-100/LConn3 -- Branch94-96/LConn3 -- Branch94-95/LConn3 -- Branch93-94/RConn3
  Branch92-100/RConn1 -- Bus100/RConn1 -- Branch100-100/LConn1 -- Branch100-106/LConn1 -- Branch100-104/LConn1 -- Branch100-103/LConn1 -- Branch100-101/LConn1 -- Branch99-100/RConn1 -- Branch98-100/RConn1 -- Branch94-100/RConn1
  Branch92-100/RConn2 -- Bus100/RConn2 -- Branch100-100/LConn2 -- Branch100-106/LConn2 -- Branch100-104/LConn2 -- Branch100-103/LConn2 -- Branch100-101/LConn2 -- Branch99-100/RConn2 -- Branch98-100/RConn2 -- Branch94-100/RConn2
  Branch92-100/RConn3 -- Bus100/RConn3 -- Branch100-100/LConn3 -- Branch100-106/LConn3 -- Branch100-104/LConn3 -- Branch100-103/LConn3 -- Branch100-101/LConn3 -- Branch99-100/RConn3 -- Branch98-100/RConn3 -- Branch94-100/RConn3
  Branch92-102/RConn1 -- Bus102/RConn1 -- Branch102-102/LConn1 -- Branch101-102/RConn1
  Branch92-102/RConn2 -- Bus102/RConn2 -- Branch102-102/LConn2 -- Branch101-102/RConn2
  Branch92-102/RConn3 -- Bus102/RConn3 -- Branch102-102/LConn3 -- Branch101-102/RConn3
  Branch94-95/RConn1 -- Bus95/RConn1 -- Branch95-95/LConn1 -- Branch95-96/LConn1
  Branch94-95/RConn2 -- Bus95/RConn2 -- Branch95-95/LConn2 -- Branch95-96/LConn2
  Branch94-95/RConn3 -- Bus95/RConn3 -- Branch95-95/LConn3 -- Branch95-96/LConn3
  Branch100-101/RConn1 -- Bus101/RConn1 -- Branch101-101/LConn1 -- Branch101-102/LConn1
  Branch100-101/RConn2 -- Bus101/RConn2 -- Branch101-101/LConn2 -- Branch101-102/LConn2
  Branch100-101/RConn3 -- Bus101/RConn3 -- Branch101-101/LConn3 -- Branch101-102/LConn3
  Branch100-103/RConn1 -- Bus103/RConn1 -- Branch103-103/LConn1 -- Branch103-110/LConn1 -- Branch103-105/LConn1 -- Branch103-104/LConn1
  Branch100-103/RConn2 -- Bus103/RConn2 -- Branch103-103/LConn2 -- Branch103-110/LConn2 -- Branch103-105/LConn2 -- Branch103-104/LConn2
  Branch100-103/RConn3 -- Bus103/RConn3 -- Branch103-103/LConn3 -- Branch103-110/LConn3 -- Branch103-105/LConn3 -- Branch103-104/LConn3
  Branch100-104/RConn1 -- Bus104/RConn1 -- Branch104-104/LConn1 -- Branch104-105/LConn1 -- Branch103-104/RConn1
  Branch100-104/RConn2 -- Bus104/RConn2 -- Branch104-104/LConn2 -- Branch104-105/LConn2 -- Branch103-104/RConn2
  Branch100-104/RConn3 -- Bus104/RConn3 -- Branch104-104/LConn3 -- Branch104-105/LConn3 -- Branch103-104/RConn3
  Branch100-106/RConn1 -- Bus106/RConn1 -- Branch106-106/LConn1 -- Branch106-107/LConn1 -- Branch105-106/RConn1
  Branch100-106/RConn2 -- Bus106/RConn2 -- Branch106-106/LConn2 -- Branch106-107/LConn2 -- Branch105-106/RConn2
  Branch100-106/RConn3 -- Bus106/RConn3 -- Branch106-106/LConn3 -- Branch106-107/LConn3 -- Branch105-106/RConn3
  Branch103-105/RConn1 -- Bus105/RConn1 -- Branch105-105/LConn1 -- Branch105-108/LConn1 -- Branch105-107/LConn1 -- Branch105-106/LConn1 -- Branch104-105/RConn1
  Branch103-105/RConn2 -- Bus105/RConn2 -- Branch105-105/LConn2 -- Branch105-108/LConn2 -- Branch105-107/LConn2 -- Branch105-106/LConn2 -- Branch104-105/RConn2
  Branch103-105/RConn3 -- Bus105/RConn3 -- Branch105-105/LConn3 -- Branch105-108/LConn3 -- Branch105-107/LConn3 -- Branch105-106/LConn3 -- Branch104-105/RConn3
  Branch103-110/RConn1 -- Bus110/RConn1 -- Branch110-110/LConn1 -- Branch110-112/LConn1 -- Branch110-111/LConn1 -- Branch109-110/RConn1
  Branch103-110/RConn2 -- Bus110/RConn2 -- Branch110-110/LConn2 -- Branch110-112/LConn2 -- Branch110-111/LConn2 -- Branch109-110/RConn2
  Branch103-110/RConn3 -- Bus110/RConn3 -- Branch110-110/LConn3 -- Branch110-112/LConn3 -- Branch110-111/LConn3 -- Branch109-110/RConn3
  Branch105-107/RConn1 -- Bus107/RConn1 -- Branch107-107/LConn1 -- Branch106-107/RConn1
  Branch105-107/RConn2 -- Bus107/RConn2 -- Branch107-107/LConn2 -- Branch106-107/RConn2
  Branch105-107/RConn3 -- Bus107/RConn3 -- Branch107-107/LConn3 -- Branch106-107/RConn3
  Branch105-108/RConn1 -- Bus108/RConn1 -- Branch108-108/LConn1 -- Branch108-109/LConn1
  Branch105-108/RConn2 -- Bus108/RConn2 -- Branch108-108/LConn2 -- Branch108-109/LConn2
  Branch105-108/RConn3 -- Bus108/RConn3 -- Branch108-108/LConn3 -- Branch108-109/LConn3
  Branch108-109/RConn1 -- Bus109/RConn1 -- Branch109-109/LConn1 -- Branch109-110/LConn1
  Branch108-109/RConn2 -- Bus109/RConn2 -- Branch109-109/LConn2 -- Branch109-110/LConn2
  Branch108-109/RConn3 -- Bus109/RConn3 -- Branch109-109/LConn3 -- Branch109-110/LConn3
  Branch110-111/RConn1 -- Bus111/RConn1 -- Branch111-111/LConn1
  Branch110-111/RConn2 -- Bus111/RConn2 -- Branch111-111/LConn2
  Branch110-111/RConn3 -- Bus111/RConn3 -- Branch111-111/LConn3
  Branch110-112/RConn1 -- Bus112/RConn1 -- Branch112-112/LConn1
  Branch110-112/RConn2 -- Bus112/RConn2 -- Branch112-112/LConn2
  Branch110-112/RConn3 -- Bus112/RConn3 -- Branch112-112/LConn3
  SM1/LConn1 -- Bus1/LConn1
  SM1/LConn2 -- Bus1/LConn2
  SM1/LConn3 -- Bus1/LConn3
  SM4/LConn1 -- Bus4/LConn1
  SM4/LConn2 -- Bus4/LConn2
  SM4/LConn3 -- Bus4/LConn3
  VSI-PLL6/LConn1 -- Bus6/LConn1
  VSI-PLL6/LConn2 -- Bus6/LConn2
  VSI-PLL6/LConn3 -- Bus6/LConn3
  SM8/LConn1 -- Bus8/LConn1
  SM8/LConn2 -- Bus8/LConn2
  SM8/LConn3 -- Bus8/LConn3
  VSI-PLL10/LConn1 -- Bus10/LConn1
  VSI-PLL10/LConn2 -- Bus10/LConn2
  VSI-PLL10/LConn3 -- Bus10/LConn3
  VSI-PLL12/LConn1 -- Bus12/LConn1
  VSI-PLL12/LConn2 -- Bus12/LConn2
  VSI-PLL12/LConn3 -- Bus12/LConn3
  SM15/LConn1 -- Bus15/LConn1
  SM15/LConn2 -- Bus15/LConn2
  SM15/LConn3 -- Bus15/LConn3
  SM18/LConn1 -- Bus18/LConn1
  SM18/LConn2 -- Bus18/LConn2
  SM18/LConn3 -- Bus18/LConn3
  VSI-PLL19/LConn1 -- Bus19/LConn1
  VSI-PLL19/LConn2 -- Bus19/LConn2
  VSI-PLL19/LConn3 -- Bus19/LConn3
  SM24/LConn1 -- Bus24/LConn1
  SM24/LConn2 -- Bus24/LConn2
  SM24/LConn3 -- Bus24/LConn3
  SM25/LConn1 -- Bus25/LConn1
  SM25/LConn2 -- Bus25/LConn2
  SM25/LConn3 -- Bus25/LConn3
  VSI-PLL26/LConn1 -- Bus26/LConn1
  VSI-PLL26/LConn2 -- Bus26/LConn2
  VSI-PLL26/LConn3 -- Bus26/LConn3
  VSI-PLL27/LConn1 -- Bus27/LConn1
  VSI-PLL27/LConn2 -- Bus27/LConn2
  VSI-PLL27/LConn3 -- Bus27/LConn3
  SM31/LConn1 -- Bus31/LConn1
  SM31/LConn2 -- Bus31/LConn2
  SM31/LConn3 -- Bus31/LConn3
  VSI-PLL32/LConn1 -- Bus32/LConn1
  VSI-PLL32/LConn2 -- Bus32/LConn2
  VSI-PLL32/LConn3 -- Bus32/LConn3
  SM34/LConn1 -- Bus34/LConn1
  SM34/LConn2 -- Bus34/LConn2
  SM34/LConn3 -- Bus34/LConn3
  SM36/LConn1 -- Bus36/LConn1
  SM36/LConn2 -- Bus36/LConn2
  SM36/LConn3 -- Bus36/LConn3
  SM40/LConn1 -- Bus40/LConn1
  SM40/LConn2 -- Bus40/LConn2
  SM40/LConn3 -- Bus40/LConn3
  VSI-PLL42/LConn1 -- Bus42/LConn1
  VSI-PLL42/LConn2 -- Bus42/LConn2
  VSI-PLL42/LConn3 -- Bus42/LConn3
  SM46/LConn1 -- Bus46/LConn1
  SM46/LConn2 -- Bus46/LConn2
  SM46/LConn3 -- Bus46/LConn3
  SM49/LConn1 -- Bus49/LConn1
  SM49/LConn2 -- Bus49/LConn2
  SM49/LConn3 -- Bus49/LConn3
  SM54/LConn1 -- Bus54/LConn1
  SM54/LConn2 -- Bus54/LConn2
  SM54/LConn3 -- Bus54/LConn3
  SM55/LConn1 -- Bus55/LConn1
  SM55/LConn2 -- Bus55/LConn2
  SM55/LConn3 -- Bus55/LConn3
  VSI-PLL56/LConn1 -- Bus56/LConn1
  VSI-PLL56/LConn2 -- Bus56/LConn2
  VSI-PLL56/LConn3 -- Bus56/LConn3
  SM59/LConn1 -- Bus59/LConn1
  SM59/LConn2 -- Bus59/LConn2
  SM59/LConn3 -- Bus59/LConn3
  SM61/LConn1 -- Bus61/LConn1
  SM61/LConn2 -- Bus61/LConn2
  SM61/LConn3 -- Bus61/LConn3
  VSI-PLL62/LConn1 -- Bus62/LConn1
  VSI-PLL62/LConn2 -- Bus62/LConn2
  VSI-PLL62/LConn3 -- Bus62/LConn3
  SM65/LConn1 -- Bus65/LConn1
  SM65/LConn2 -- Bus65/LConn2
  SM65/LConn3 -- Bus65/LConn3
  VSI-PLL66/LConn1 -- Bus66/LConn1
  VSI-PLL66/LConn2 -- Bus66/LConn2
  VSI-PLL66/LConn3 -- Bus66/LConn3
  SM69/LConn1 -- Bus69/LConn1
  SM69/LConn2 -- Bus69/LConn2
  SM69/LConn3 -- Bus69/LConn3
  VSI-PLL70/LConn1 -- Bus70/LConn1
  VSI-PLL70/LConn2 -- Bus70/LConn2
  VSI-PLL70/LConn3 -- Bus70/LConn3
  SM72/LConn1 -- Bus72/LConn1
  SM72/LConn2 -- Bus72/LConn2
  SM72/LConn3 -- Bus72/LConn3
  SM73/LConn1 -- Bus73/LConn1
  SM73/LConn2 -- Bus73/LConn2
  SM73/LConn3 -- Bus73/LConn3
  VSI-PLL74/LConn1 -- Bus74/LConn1
  VSI-PLL74/LConn2 -- Bus74/LConn2
  VSI-PLL74/LConn3 -- Bus74/LConn3
  SM76/LConn1 -- Bus76/LConn1
  SM76/LConn2 -- Bus76/LConn2
  SM76/LConn3 -- Bus76/LConn3
  VSI-PLL77/LConn1 -- Bus77/LConn1
  VSI-PLL77/LConn2 -- Bus77/LConn2
  VSI-PLL77/LConn3 -- Bus77/LConn3
  SM80/LConn1 -- Bus80/LConn1
  SM80/LConn2 -- Bus80/LConn2
  SM80/LConn3 -- Bus80/LConn3
  VSI-PLL85/LConn1 -- Bus85/LConn1
  VSI-PLL85/LConn2 -- Bus85/LConn2
  VSI-PLL85/LConn3 -- Bus85/LConn3
  SM87/LConn1 -- Bus87/LConn1
  SM87/LConn2 -- Bus87/LConn2
  SM87/LConn3 -- Bus87/LConn3
  SM89/LConn1 -- Bus89/LConn1
  SM89/LConn2 -- Bus89/LConn2
  SM89/LConn3 -- Bus89/LConn3
  SM90/LConn1 -- Bus90/LConn1
  SM90/LConn2 -- Bus90/LConn2
  SM90/LConn3 -- Bus90/LConn3
  VSI-PLL91/LConn1 -- Bus91/LConn1
  VSI-PLL91/LConn2 -- Bus91/LConn2
  VSI-PLL91/LConn3 -- Bus91/LConn3
  VSI-PLL92/LConn1 -- Bus92/LConn1
  VSI-PLL92/LConn2 -- Bus92/LConn2
  VSI-PLL92/LConn3 -- Bus92/LConn3
  SM99/LConn1 -- Bus99/LConn1
  SM99/LConn2 -- Bus99/LConn2
  SM99/LConn3 -- Bus99/LConn3
  SM100/LConn1 -- Bus100/LConn1
  SM100/LConn2 -- Bus100/LConn2
  SM100/LConn3 -- Bus100/LConn3
  SM103/LConn1 -- Bus103/LConn1
  SM103/LConn2 -- Bus103/LConn2
  SM103/LConn3 -- Bus103/LConn3
  SM104/LConn1 -- Bus104/LConn1
  SM104/LConn2 -- Bus104/LConn2
  SM104/LConn3 -- Bus104/LConn3
  VSI-PLL105/LConn1 -- Bus105/LConn1
  VSI-PLL105/LConn2 -- Bus105/LConn2
  VSI-PLL105/LConn3 -- Bus105/LConn3
  SM107/LConn1 -- Bus107/LConn1
  SM107/LConn2 -- Bus107/LConn2
  SM107/LConn3 -- Bus107/LConn3
  SM110/LConn1 -- Bus110/LConn1
  SM110/LConn2 -- Bus110/LConn2
  SM110/LConn3 -- Bus110/LConn3
  SM111/LConn1 -- Bus111/LConn1
  SM111/LConn2 -- Bus111/LConn2
  SM111/LConn3 -- Bus111/LConn3
  VSI-PLL112/LConn1 -- Bus112/LConn1
  VSI-PLL112/LConn2 -- Bus112/LConn2
  VSI-PLL112/LConn3 -- Bus112/LConn3
  VSI-PLL113/LConn1 -- Bus113/LConn1
  VSI-PLL113/LConn2 -- Bus113/LConn2
  VSI-PLL113/LConn3 -- Bus113/LConn3
  VSI-PLL116/LConn1 -- Bus116/LConn1
  VSI-PLL116/LConn2 -- Bus116/LConn2
  VSI-PLL116/LConn3 -- Bus116/LConn3
  B-GND2/LConn1 -- Load Step/RConn1
  Load Step/LConn1 -- Bus68/LConn1
  Load Step/LConn2 -- Bus68/LConn2
  Load Step/LConn3 -- Bus68/LConn3
